simulink model "Model_Reduction_Scaling_Observer_Stable"  (R2021a)
settings: Solver=ode1  StartTime=0.0  StopTime=20  FixedStep=0.0001  RelTol=1e-3
values from neighbouring files (symbols this model uses):
  A = [zeros(8),eye(8);-inv(M)*(Ks+Kus),-inv(M)*(CA+CD)]    [Bogie_ModelReduction_Scaling_Stable.m]    (also in Eigenvalue_A_Stable.m)
  A_r = sysdel.A    [Bogie_ModelReduction_Scaling_Stable.m]    (also in Eigenvalue_A_Stable.m)
  B_r = B_r_ext(:,1:2)    [Bogie_ModelReduction_Scaling_Stable.m]    (also in Eigenvalue_A_Stable.m = B_r(:,1:2))
  Bo = B    [Bogie_ModelReduction_Scaling_Stable.m]    (also in Eigenvalue_A_Stable.m)
  C = [eye(p),zeros(p,q)]    [Bogie_ModelReduction_Scaling_Stable.m]    (also in Eigenvalue_A_Stable.m)
  C_r = sysdel.C    [Bogie_ModelReduction_Scaling_Stable.m]    (also in Eigenvalue_A_Stable.m)
  L = place(A_r',C_r',poles)'    [Bogie_ModelReduction_Scaling_Stable.m]
  x_o = a*ones(16,1)    [Bogie_ModelReduction_Scaling_Stable.m]    (also in Eigenvalue_A_Stable.m)
  x_r = Tr*x_o    [Bogie_ModelReduction_Scaling_Stable.m]    (also in Eigenvalue_A_Stable.m = Ti*x_o)
undefined symbols (not defined in the file or in its folder): K1
settings Model: Creator=94503  LastModifiedBy=anniz2021
settings SolverCC: AlgebraicLoopSolver=TrustRegion
settings DebuggingCC: SFMachineParentedDataDiag=warning

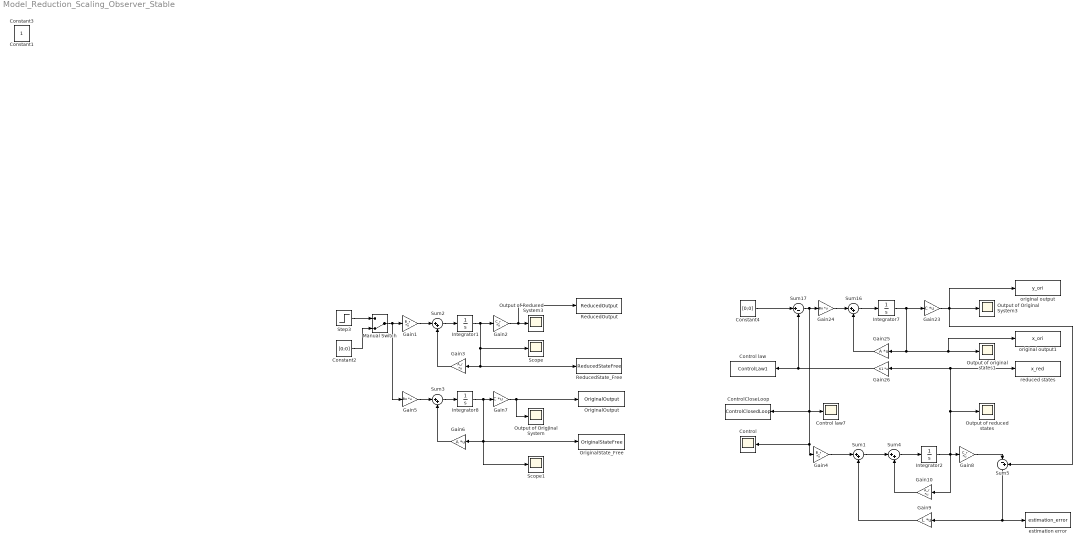
== system Model_Reduction_Scaling_Observer_Stable ==
  Constant2 : Constant  Value=[0;0]  SampleTime=0.1
  Constant4 : Constant  Value=[0;0]  SampleTime=0.1
  "Control " : Scope
  Control law : ToWorkspace  VariableName=ControlLaw1  SampleTime=-1
      settings: Save2DSignal=2-D array (concatenate along first dimension)
  Control law7 : Scope
  ControlCloseLoop : ToWorkspace  VariableName=ControlClosedLoop  SampleTime=-1
      settings: Save2DSignal=2-D array (concatenate along first dimension)
  Gain1 : Gain  Gain=B_r  Multiplication=Matrix(K*u) (u vector)
  Gain10 : Gain  Gain=A_r  Multiplication=Matrix(K*u) (u vector)
  Gain2 : Gain  Gain=C_r  Multiplication=Matrix(K*u) (u vector)
  Gain23 : Gain  Gain=C  Multiplication=Matrix(K*u) (u vector)
  Gain24 : Gain  Gain=Bo  Multiplication=Matrix(K*u) (u vector)
  Gain25 : Gain  Gain=A  Multiplication=Matrix(K*u) (u vector)
  Gain26 : Gain  Gain=K1  Multiplication=Matrix(K*u)
  Gain3 : Gain  Gain=A_r  Multiplication=Matrix(K*u) (u vector)
  Gain4 : Gain  Gain=B_r  Multiplication=Matrix(K*u) (u vector)
  Gain5 : Gain  Gain=Bo  Multiplication=Matrix(K*u) (u vector)
  Gain6 : Gain  Gain=A  Multiplication=Matrix(K*u) (u vector)
  Gain7 : Gain  Gain=C  Multiplication=Matrix(K*u) (u vector)
  Gain8 : Gain  Gain=C_r  Multiplication=Matrix(K*u) (u vector)
  Gain9 : Gain  Gain=L  Multiplication=Matrix(K*u) (u vector)
  Integrator1 : Integrator  InitialCondition=x_r
  Integrator2 : Integrator  InitialCondition=x_r
  Integrator7 : Integrator  InitialCondition=x_o
  Integrator8 : Integrator  InitialCondition=x_o
  Manual Switch : ManualSwitch  CurrentSetting=0
  OriginalOutput : ToWorkspace  VariableName=OriginalOutput  SampleTime=-1
      settings: Save2DSignal=2-D array (concatenate along first dimension)
  OriginalState_Free : ToWorkspace  VariableName=OriginalStateFree  SampleTime=-1
      settings: Save2DSignal=2-D array (concatenate along first dimension)
  Output of Original System3 : Scope
  Output of Origjinal System : Scope
  Output of Reduced System3 : Scope
  Output of original states1 : Scope
  Output of reduced states : Scope
  ReducedOutput : ToWorkspace  VariableName=ReducedOutput  SampleTime=-1
      settings: Save2DSignal=2-D array (concatenate along first dimension)
  ReducedState_Free : ToWorkspace  VariableName=ReducedStateFree  SampleTime=-1
      settings: Save2DSignal=2-D array (concatenate along first dimension)
  Scope : Scope
  Scope1 : Scope
  Step3 : Step  Time=[1;1]  SampleTime=0.01
  Sum{1..4,16} (5 alike) : Sum  Inputs=|++
  Sum17 : Sum  Inputs=|+-
  Sum5 : Sum  Inputs=|-+
  estimation error : ToWorkspace  VariableName=estimation_error  SampleTime=-1
      settings: Save2DSignal=2-D array (concatenate along first dimension)
  original output : ToWorkspace  VariableName=y_ori  SampleTime=-1
      settings: Save2DSignal=2-D array (concatenate along first dimension)
  original output1 : ToWorkspace  VariableName=x_ori  SampleTime=-1
      settings: Save2DSignal=2-D array (concatenate along first dimension)
  reduced states : ToWorkspace  VariableName=x_red  SampleTime=-1
      settings: Save2DSignal=2-D array (concatenate along first dimension)
  Constant1 : Constant  IOType=siggen
  Constant3 : Constant  IOType=siggen
  wires:
  Integrator7/1 -> Output of original states1/1, original output1/1, Gain25/1, Gain23/1
  Gain25/1 -> Sum16/2
  Gain24/1 -> Sum16/1
  Sum17/1 -> "Control "/1, Gain4/1, Control law7/1, ControlCloseLoop/1, Gain24/1
  Constant4/1 -> Sum17/1
  Sum16/1 -> Integrator7/1
  Gain23/1 -> Sum5/2, original output/1, Output of Original System3/1
  Gain3/1 -> Sum2/2
  Gain1/1 -> Sum2/1
  Integrator1/1 -> Gain3/1, ReducedState_Free/1, Scope/1, Gain2/1
  Sum2/1 -> Integrator1/1
  Gain2/1 -> ReducedOutput/1, Output of Reduced System3/1
  Gain6/1 -> Sum3/2
  Integrator8/1 -> Gain7/1, Scope1/1, Gain6/1, OriginalState_Free/1
  Sum3/1 -> Integrator8/1
  Gain5/1 -> Sum3/1
  Gain4/1 -> Sum1/1
  Sum1/1 -> Sum4/1
  Sum4/1 -> Integrator2/1
  Integrator2/1 -> Gain10/1, Gain26/1, reduced states/1, Output of reduced states/1, Gain8/1
  Gain8/1 -> Sum5/1
  Gain10/1 -> Sum4/2
  Sum5/1 -> Gain9/1, estimation error/1
  Gain9/1 -> Sum1/2
  Gain26/1 -> Control law/1, Sum17/2
  Gain7/1 -> Output of Origjinal System/1, OriginalOutput/1
  Step3/1 -> Manual Switch/1
  Constant2/1 -> Manual Switch/2
  Manual Switch/1 -> Gain1/1, Gain5/1
